simulink model "sim_aut_dual_scen"  (R2025b)
settings: Solver=ode45  StartTime=0.0  StopTime=Tfin  FixedStep=1e-3  MaxStep=1e-2  MinStep=1e-3  RelTol=5e-3
values from neighbouring files (symbols this model uses):
  bp = [-1.25 -1.19897959184 -1.14795918367 -1.09693877551 -1.04591836735 -0.994897959184 -0.94387755102 -0.892857142857 -0.841836734694 -0.790816326531 -0.739795918367 -0.688775510204 ... (50 elements, 1x50)]    [tire_model.mat]
  C1 = 2.7e4    (= 27000)    [main.m]    (also in model.m)
  C2 = 2e4    (= 20000)    [main.m]    (also in model.m)
  Jz = 4000    [main.m]    (also in model.m)
  K = nmpc_design_st2(par,2)    [main.m]
  l1 = 1.2    [main.m]    (also in model.m)
  l2 = 1.6    [main.m]    (also in model.m)
  m = 1575    [main.m]    (also in model.m)
  Np = round(vx_ref*K.Tp/mean(ds))    [main.m]
  pacf = [2550.90487699 2674.70463742 2810.77279096 2960.97362657 3127.55760929 3313.26346728 3521.4532226 3756.29269015 4022.99538347 4328.15571957 4680.20907939 5090.07319782 ... (50 elements, 1x50)]    [tire_model.mat]
  pacr = [2550.90487699 2674.70463742 2810.77279096 2960.97362657 3127.55760929 3313.26346728 3521.4532226 3756.29269015 4022.99538347 4328.15571957 4680.20907939 5090.07319782 ... (50 elements, 1x50)]    [tire_model.mat]
  psi = x(3)    [model.m]
  psir = [atan2(diff(Yr),diff(Xr));0]    [main.m]
  refPoses = [Xr,Yr,psir]    [main.m]
  Ts = 0.05    [main.m]
  ze0 = [X0;Y0;psi0;vx0;vy0;wpsi0]    [main.m]
undefined symbols (not defined in the file or in its folder): aMode, plot_ref, x_o
libraries: autolibsharedcommon x11, autolibshared x5, autolibpowerinfoutils x2, autolibutils x2, sharedtransform x2, simulink x1, drivingscenarioandsensors x1
(part 4 of 4)

== matlab function sim_aut_dual_scen/reference generator1/Subsystem/errors/MATLAB Function ==
  data: e_y_dot output; ref input; psi_r_dot input; e_psi output; e_psi_dot output; ze input
function [e_y_dot,e_psi,e_psi_dot]=errors(ref,psi_r_dot,ze)

e_psi=ze(3)-ref(3);
e_psi_dot=ze(6)-psi_r_dot;
e_y_dot=ze(5)+ze(4)*e_psi;

== matlab function sim_aut_dual_scen/vehicle/dual-track/Vehicle Body 3DOF Dual Track/Signal Routing/Signal Routing/state2bus/COMB2I ==
  data: x input size=4; y output size=2
function y = fcn(x)%#codegen
coder.allowpcode('plain')
y = automlvehb2i(x);

== matlab function sim_aut_dual_scen/vehicle/dual-track/Vehicle Body 3DOF Dual Track/Signal Routing/Signal Routing Dual/state2bus/COMB2I ==
  data: x input size=4; y output size=2
function y = fcn(x)%#codegen
coder.allowpcode('plain')
y = automlvehb2i(x);
